simulink model "control_PD"  (R2022b)
settings: Solver=VariableStepAuto  StartTime=0.0  StopTime=200  RelTol=1e-3
libraries: fuzblock x1
settings Model: Creator=sophy  LastModifiedBy=sophy

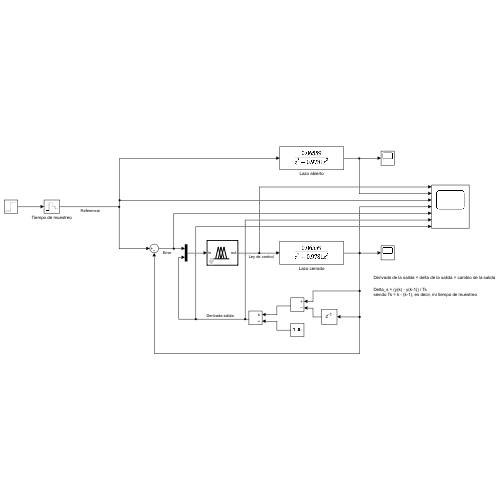
[thumbnail: Simulink's stored preview of the top-level diagram]
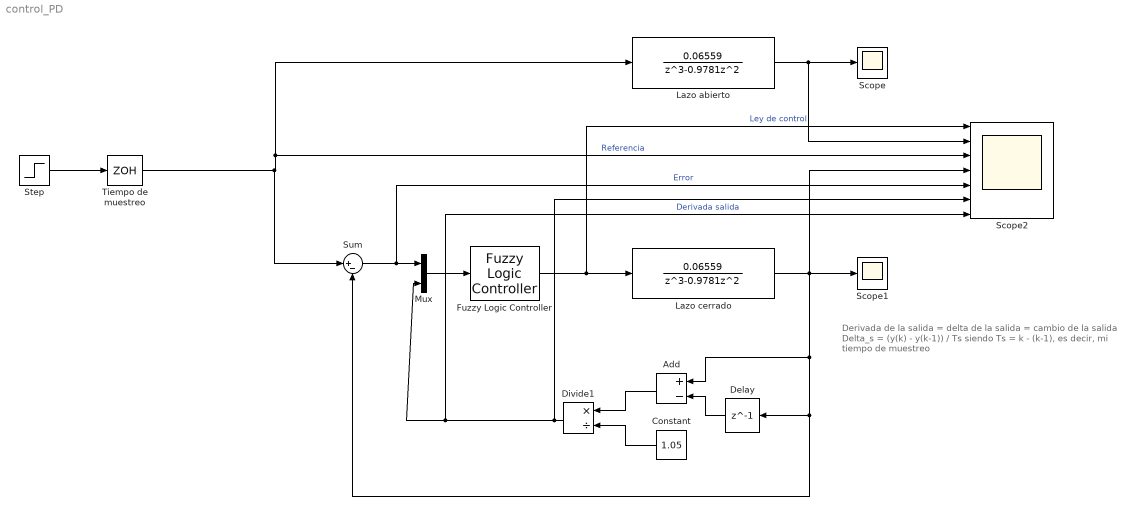
== system control_PD ==
  note: Derivada de la salida = delta de la salida = cambio de la salida
      |
      | Delta_s = (y(k) - y(k-1)) / Ts
      | siendo Ts = k - (k-1), es decir, mi tiempo de muestreo
  Add : Sum  Inputs=+-
  Constant : Constant  Value=1.05
  Delay : Delay  DelayLength=1
  Divide1 : Product  Inputs=*/
  Fuzzy Logic Controller : fuzblock/Fuzzy Logic  Controller  FIS=control_PD  OutputSampleNumber=101  DataType=double  FuzzifiedInputs=off  RuleFiringStrengths=off  RuleOutputs=off  AggregatedOutputs=off  SimulateUsing=Interpreted execution  OutOfRangeInputValueMessage=warning  NoRuleFiredMessage=warning  EmptyOutputFuzzySetMessage=warning
  Lazo abierto : DiscreteTransferFcn  Numerator=[0.06559]  Denominator=[1 -0.9781 0 0]
  Lazo cerrado : DiscreteTransferFcn  Numerator=[0.06559]  Denominator=[1 -0.9781 0 0]
  Mux : Mux  Inputs=2
  Scope : Scope
  Scope1 : Scope
  Scope2 : Scope  NumInputPorts=7
  Step : Step  After=10  SampleTime=0
  Sum : Sum  Inputs=|+-
  Tiempo de muestreo : ZeroOrderHold  SampleTime=1.05
  wires:
  Mux/1 -> Fuzzy Logic Controller/1
  Divide1/1 -> Scope2/6, Mux/2, Scope2/7  "Derivada salida"
  Constant/1 -> Divide1/2
  Lazo cerrado/1 -> Add/1, Delay/1, Sum/2, Scope2/4, Scope1/1
  Sum/1 -> Scope2/5, Mux/1  "Error"
  Delay/1 -> Add/2
  Tiempo de muestreo/1 -> Sum/1, Lazo abierto/1, Scope2/3  "Referencia"
  Lazo abierto/1 -> Scope/1, Scope2/2
  Add/1 -> Divide1/1
  Fuzzy Logic Controller/1 -> Lazo cerrado/1, Scope2/1  "Ley de control"
  Step/1 -> Tiempo de muestreo/1
